simulink library "My_library"  (R2024b)
settings: Solver=VariableStepAuto  StartTime=0.0  StopTime=10.0  RelTol=1e-3
undefined symbols (not defined in the file): DiscIntNeverNeededParam, L
libraries: slpidlib x3, dspfdesign x2, eeGeneralControl x1
settings Model: Creator=sa127  LastModifiedBy=sa127

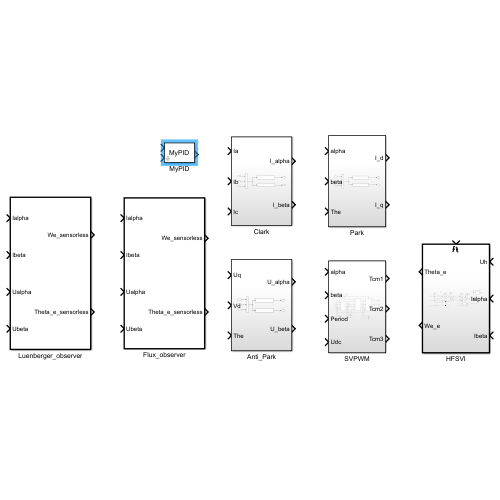
[thumbnail: Simulink's stored preview of the top-level diagram]
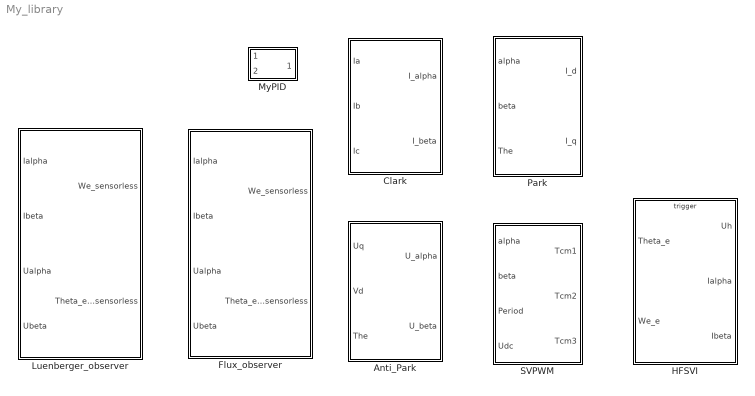
== system My_library ==
  Anti_Park : Subsystem
  Clark : Subsystem
  Flux_observer : Subsystem  TreatAsAtomicUnit=on  mask{gamma=100000, PLL_P=0, PLL_I=0, Rs=0, Ls=0, flux=0, Ts=0}
      mask prompts: gamma "磁链观测器增益"; PLL_P "锁相环Kp"; PLL_I "锁相环Ki"; Rs "电机相电阻"; Ls "电机相电感"; flux "永磁体磁链"; Ts "计算周期"
      mask DialogControl ParameterGroupVar Prompt: 参数
  HFSVI : Subsystem  TreatAsAtomicUnit=on
  Luenberger_observer : Subsystem  TreatAsAtomicUnit=on  mask{Rs=0, Ls=0, K1=0, K2=0, PLL_P=0, PLL_I=0, Ts=0}
      mask prompts: Rs "电机相电阻"; Ls "电机相电感"; K1 "增益K1"; K2 "增益K2"; PLL_P "锁相环Kp"; PLL_I "锁相环Ki"; Ts "运行周期"
      mask DialogControl ParameterGroupVar Prompt: 参数
  MyPID : Subsystem  mask{Kp=0.05, Ki=5, Kd=0, Ts=0.0001, max_Integral=500, min_Integral=-500, max_output=500, min_output=-500}
      mask prompts: max_Integral "积分上限"; min_Integral "积分下限"; max_output "输出上限"; min_output "输出下限"
      mask DialogControl DescTextVar Prompt: PID控制器
      mask DialogControl ParameterGroupVar Prompt: 参数
      mask Display: fprintf('MyPID');
  Park : Subsystem
  SVPWM : Subsystem

== system My_library/Anti_Park ==
  Uq : Inport
  Vd : Inport  Port=2
  The : Inport  Port=3
  Fcn : Fcn  Expr=cos(u(3))*u(2)-sin(u(3))*u(1)
  Fcn1 : Fcn  Expr=sin(u(3))*u(2)+cos(u(3))*u(1)
  Mux : Mux  Inputs=3
  U_alpha : Outport
  U_beta : Outport  Port=2
  wires:
  The/1 -> Mux/3
  Uq/1 -> Mux/1
  Fcn1/1 -> U_beta/1
  Vd/1 -> Mux/2
  Fcn/1 -> U_alpha/1
  Mux/1 -> Fcn/1, Fcn1/1

== system My_library/Clark ==
  Ia : Inport
  Ib : Inport  Port=2
  Ic : Inport  Port=3
  Fcn : Fcn  Expr=(u(1)-0.5*u(2)-0.5*u(3))*2/3
  Fcn1 : Fcn  Expr=(sqrt(3)/2*u(2)-sqrt(3)/2*u(3))*2/3
  Mux : Mux  Inputs=3
  I_alpha : Outport
  I_beta : Outport  Port=2
  wires:
  Ia/1 -> Mux/1
  Fcn/1 -> I_alpha/1
  Mux/1 -> Fcn/1, Fcn1/1
  Ic/1 -> Mux/3
  Fcn1/1 -> I_beta/1
  Ib/1 -> Mux/2

== system My_library/Flux_observer ==
  Ialpha : Inport
  Ibeta : Inport  Port=2
  Ualpha : Inport  Port=3
  Ubeta : Inport  Port=4
  OBSERVER : Subsystem
  PLL : Subsystem
  Scope6 : Scope  NumInputPorts=2
  We_sensorless : Outport
  Theta_e_sensorless : Outport  Port=2
  wires:
  Ibeta/1 -> OBSERVER/2(Ibeta)
  OBSERVER/1(sin) -> PLL/1(sin), Scope6/1  "sin_theta"
  OBSERVER/2(cos) -> PLL/2(cos), Scope6/2  "cos_theta"
  PLL/1(We) -> We_sensorless/1
  PLL/2(Theta_e) -> Theta_e_sensorless/1
  Ualpha/1 -> OBSERVER/3(Ualpha)
  Ubeta/1 -> OBSERVER/4(Ubeta)
  Ialpha/1 -> OBSERVER/1(Ialpha)

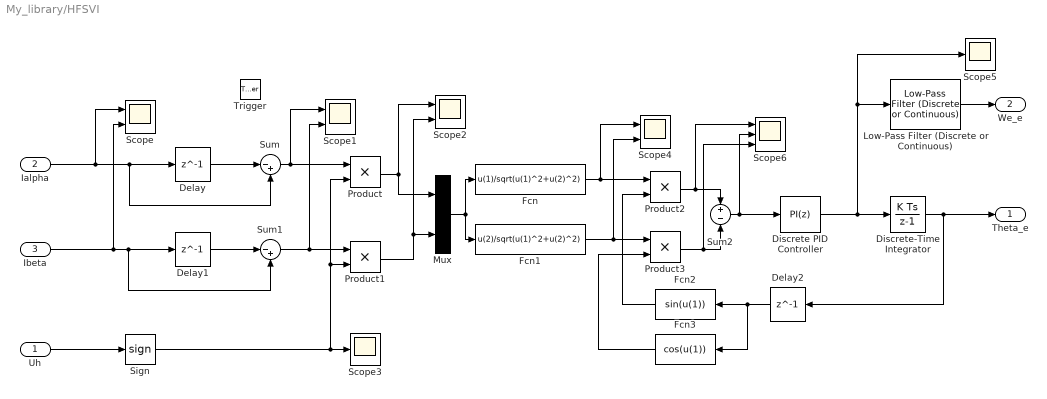
== system My_library/HFSVI ==
  Uh : Inport
  Ialpha : Inport  Port=2
  Ibeta : Inport  Port=3
  Trigger : TriggerPort  TriggerType=either  VariantControl=(inherit)
  Delay : Delay  DelayLength=1  InitialCondition=0
  Delay1 : Delay  DelayLength=1  InitialCondition=0
  Delay2 : Delay  DelayLength=1  InitialCondition=0
  Discrete PID Controller : slpidlib/PID Controller  Controller=PI  Form=Parallel  TimeDomain=Discrete-time  UseExternalTs=off  SampleTime=-1  IntegratorMethod=Forward Euler  FilterMethod=Forward Euler  ControllerParametersSource=internal  P=300  I=40000  UseKiTs=off  D=0  UseExternalDerivativeSource=off  N=100  UseFilter=on  TunerSelectOption=Transfer Function Based (PID Tuner App)  InitialConditionSource=internal  InitialConditionForIntegrator=0  InitialConditionForFilter=0  DifferentiatorICPrevScaledInput=0  ExternalReset=none  TrackingMode=off  Kt=1  LimitOutput=off  SatLimitsSource=internal  UpperSaturationLimit=inf  LowerSaturationLimit=-inf  LinearizeAsGain=off  AntiWindupMode=none  Kb=1  LimitIntegrator=off  UpperIntegratorSaturationLimit=inf  LowerIntegratorSaturationLimit=-inf  POutMin=[]  POutMax=[]  IOutMin=[]  IOutMax=[]  DOutMin=[]  DOutMax=[]  NOutMin=[]  NOutMax=[]  SumOutMin=[]  SumOutMax=[]  SaturationOutMin=[]  SaturationOutMax=[]  PParamMin=[]  PParamMax=[]  IParamMin=[]  IParamMax=[]  DParamMin=[]  DParamMax=[]  NParamMin=[]  NParamMax=[]  KbParamMin=[]  KbParamMax=[]  KtParamMin=[]  KtParamMax=[]  KbOutMin=[]  KbOutMax=[]  KtOutMin=[]  KtOutMax=[]  IntegratorOutMin=[]  IntegratorOutMax=[]  FilterOutMin=[]  FilterOutMax=[]  SumI1OutMin=[]  SumI1OutMax=[]  SumI2OutMin=[]  SumI2OutMax=[]  SumI3OutMin=[]  SumI3OutMax=[]  SumI4OutMin=[]  SumI4OutMax=[]  SumDOutMin=[]  SumDOutMax=[]  DifferentiatorOutMin=[]  DifferentiatorOutMax=[]  FilterDiffOutCoefMin=[]  FilterDiffOutCoefMax=[]  ReciprocalOutMin=[]  ReciprocalOutMax=[]  SumDenOutMin=[]  SumDenOutMax=[]  SumNumOutMin=[]  SumNumOutMax=[]  DivideOutMin=[]  DivideOutMax=[]  UdiffTsProdOutMin=[]  UdiffTsProdOutMax=[]  NTsProdOutMin=[]  NTsProdOutMax=[]  UintegralTsProdOutMin=[]  UintegralTsProdOutMax=[]  UngainTsProdOutMin=[]  UngainTsProdOutMax=[]  ClampingZeroOutDataTypeStr=Inherit: Inherit via back propagation  ClampingZeroOutMin=[]  ClampingZeroOutMax=[]  FilterDenConstantOutDataTypeStr=Inherit: Inherit via back propagation  FilterDenConstantOutMin=[]  FilterDenConstantOutMax=[]  PCopyOutDataTypeStr=Inherit: Inherit via back propagation  PCopyOutMin=[]  PCopyOutMax=[]  NCopyOutDataTypeStr=Inherit: Inherit via back propagation  NCopyOutMin=[]  NCopyOutMax=[]  IntegratorContinuousStateAttributes=''  IntegratorStateMustResolveToSignalObject=off  IntegratorRTWStateStorageClass=Auto  FilterContinuousStateAttributes=''  FilterStateMustResolveToSignalObject=off  FilterRTWStateStorageClass=Auto  ParallelPVariant=InternalParameters  IdealPVariant=Disabled  IVariant=InternalParameters  DVariant=Disabled  IntegratorVariant=Discrete  SatVariant=Disabled  AWVariant=Passthrough  PCopyVariant=Disabled  TRVariant=Disabled  FdbkBlocksVariant=Forward  IdealPFdbkVariant=Disabled  SatFdbkVariant=Disabled  DerivativeFilterVariant=Disabled  NVariant=Disabled  NCopyVariant=Disabled_SignalSpec  FilterICVariant=Disabled  IntegratorICVariant=InternalICs  ExternalResetVariant=Disabled  TRSumVariant=Passthrough  SumFdbkVariant=Disabled  SumVariant=Sum_PI  TsampFilterVariant=InternalTs  TsampNgainVariant=Passthrough  TsampIntegralVariant=Disabled_SignalSpec  ExternalSaturationOutDataTypeStr=Inherit: Same as second input  DerivativeSourceVariant=Disabled  PreIntVariant=InternalPreInt
  Discrete-Time Integrator : DiscreteIntegrator  SampleTime=-1  ICPrevOutput=DiscIntNeverNeededParam  ICPrevScaledInput=DiscIntNeverNeededParam
  Fcn : Fcn  Expr=u(1)/sqrt(u(1)^2+u(2)^2)
  Fcn1 : Fcn  Expr=u(2)/sqrt(u(1)^2+u(2)^2)
  Fcn2 : Fcn  Expr=sin(u(1))
  Fcn3 : Fcn  Expr=cos(u(1))
  Low-Pass Filter (Discrete or Continuous) : eeGeneralControl/Low-Pass Filter (Discrete or Continuous)  K=1  T=0.01  B=inf  A=-inf  init_option=Inherited from block input  x0=0  Ts=-1
  Mux : Mux  Inputs=2
  Product{,1..3} (4 alike) : Product
  Scope{,1..2,4} (4 alike) : Scope  NumInputPorts=2
  Scope3 : Scope
  Scope5 : Scope
  Scope6 : Scope  NumInputPorts=3
  Sign : Signum
  Sum : Sum  Inputs=|-+
  Sum1 : Sum  Inputs=|-+
  Sum2 : Sum  Inputs=+-
  Theta_e : Outport
  We_e : Outport  Port=2
  wires:
  Delay/1 -> Sum/1
  Delay1/1 -> Sum1/1
  Sum/1 -> Product/1, Scope1/1
  Sum1/1 -> Product1/1, Scope1/2
  Uh/1 -> Sign/1
  Sign/1 -> Scope3/1, Product1/2, Product/2
  Product/1 -> Mux/1, Scope2/1
  Product1/1 -> Mux/2, Scope2/2
  Mux/1 -> Fcn1/1, Fcn/1
  Fcn/1 -> Product2/1, Scope4/1
  Fcn1/1 -> Scope4/2, Product3/1
  Fcn2/1 -> Product2/2
  Fcn3/1 -> Product3/2
  Product2/1 -> Scope6/1, Sum2/1
  Product3/1 -> Sum2/2, Scope6/3
  Discrete PID Controller/1 -> Scope5/1, Low-Pass Filter (Discrete or Continuous)/1, Discrete-Time Integrator/1
  Delay2/1 -> Fcn3/1, Fcn2/1
  Sum2/1 -> Scope6/2, Discrete PID Controller/1
  Low-Pass Filter (Discrete or Continuous)/1 -> We_e/1
  Ialpha/1 -> Sum/2, Delay/1, Scope/1
  Ibeta/1 -> Scope/2, Sum1/2, Delay1/1
  Discrete-Time Integrator/1 -> Theta_e/1, Delay2/1

== system My_library/Luenberger_observer ==
  Ialpha : Inport
  Ibeta : Inport  Port=2
  Ualpha : Inport  Port=3
  Ubeta : Inport  Port=4
  OBSERVER : Subsystem
  PLL : Subsystem
  Scope6 : Scope  NumInputPorts=2
  We_sensorless : Outport
  Theta_e_sensorless : Outport  Port=2
  wires:
  Ibeta/1 -> OBSERVER/2(Ibeta)
  OBSERVER/1(Ealpha_hat) -> PLL/1(Ealpha_hat), Scope6/1  "sin_theta"
  OBSERVER/2(Ebeta_hat) -> PLL/2(Ebeta_hat), Scope6/2  "cos_theta"
  PLL/1(We) -> We_sensorless/1, OBSERVER/5(We)
  PLL/2(Theta_e) -> Theta_e_sensorless/1
  Ualpha/1 -> OBSERVER/3(Ualpha)
  Ubeta/1 -> OBSERVER/4(Ubeta)
  Ialpha/1 -> OBSERVER/1(Ialpha)

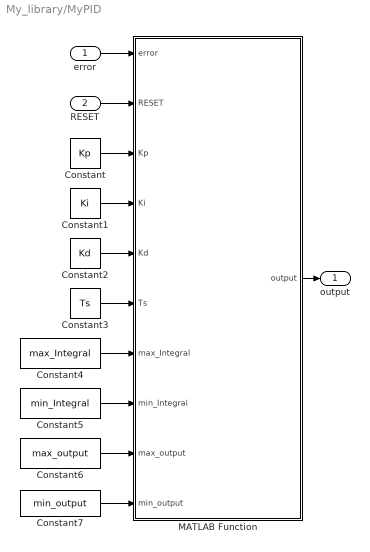
== system My_library/MyPID ==
  error : Inport
  RESET : Inport  Port=2
  Constant : Constant  Value=Kp
  Constant1 : Constant  Value=Ki
  Constant2 : Constant  Value=Kd
  Constant3 : Constant  Value=Ts
  Constant4 : Constant  Value=max_Integral
  Constant5 : Constant  Value=min_Integral
  Constant6 : Constant  Value=max_output
  Constant7 : Constant  Value=min_output
  MATLAB Function : MATLAB Function  TreatAsAtomicUnit=on
  output : Outport
  wires:
  MATLAB Function/1(output) -> output/1
  Constant2/1 -> MATLAB Function/5(Kd)
  Constant6/1 -> MATLAB Function/9(max_output)
  Constant1/1 -> MATLAB Function/4(Ki)
  error/1 -> MATLAB Function/1(error)
  Constant5/1 -> MATLAB Function/8(min_Integral)
  Constant4/1 -> MATLAB Function/7(max_Integral)
  Constant/1 -> MATLAB Function/3(Kp)
  Constant7/1 -> MATLAB Function/10(min_output)
  Constant3/1 -> MATLAB Function/6(Ts)
  RESET/1 -> MATLAB Function/2(RESET)

== system My_library/Park ==
  alpha : Inport
  beta : Inport  Port=2
  The : Inport  Port=3
  Fcn : Fcn  Expr=cos(u(3))*u(1)+sin(u(3))*u(2)
  Fcn1 : Fcn  Expr=-sin(u(3))*u(1)+cos(u(3))*u(2)
  Mux : Mux  Inputs=3
  I_d : Outport
  I_q : Outport  Port=2
  wires:
  beta/1 -> Mux/2
  Mux/1 -> Fcn/1, Fcn1/1
  alpha/1 -> Mux/1
  The/1 -> Mux/3
  Fcn1/1 -> I_q/1
  Fcn/1 -> I_d/1

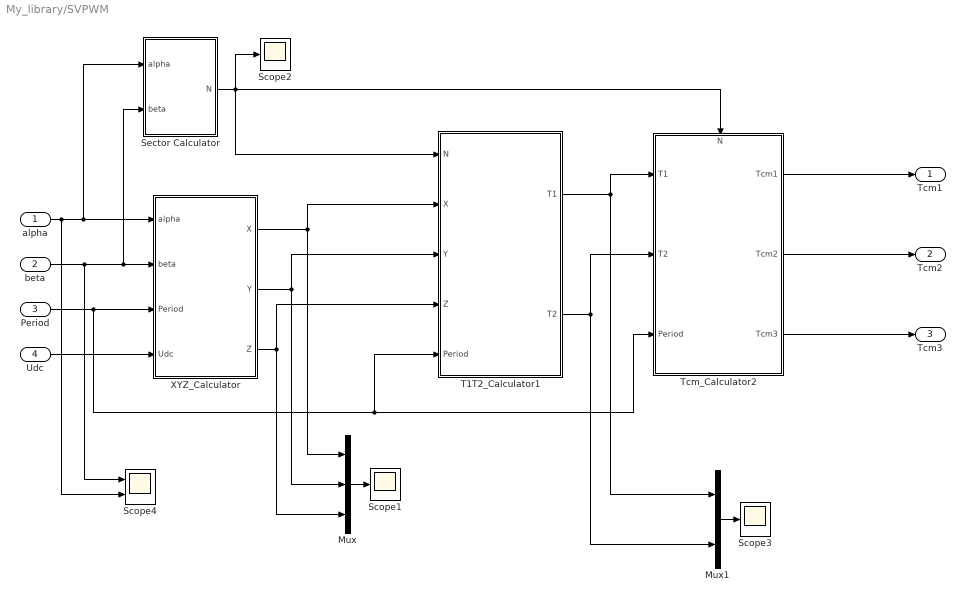
== system My_library/SVPWM ==
  alpha : Inport
  beta : Inport  Port=2
  Period : Inport  Port=3
  Udc : Inport  Port=4
  Mux : Mux  Inputs=3
  Mux1 : Mux  Inputs=2
  Scope1 : Scope
  Scope2 : Scope
  Scope3 : Scope
  Scope4 : Scope  NumInputPorts=2
  Sector Calculator : Subsystem
  T1T2_Calculator1 : Subsystem
  Tcm_Calculator2 : Subsystem
      settings: PortSchema="{\"entries\":[{\"content\":{\"sides\":[{\"content\":{\"connectorIds\":[\"In1\",\"In2\",\"In3\"]},\"type\":\"ConnectorPlacement.EquallySpacedRectSide\",\"uuid\":\"6148b169-7250-44a2-b567-24c78ff320ed\"},{\"content\":{\"connectorIds\":[\"Out1\",\"Out2\",\"Out3\"],\"side\":\"RIGHT\"},\"type\":\"ConnectorPlacement.EquallySpacedRectSide\",\"uuid\":\"6efb5841-0c91-46f1-a519-7a6c3f211abe\"},{\"content\":{\"connectorIds\":[\"In4\"],\"side\":\"TOP\"},\"type\":\"ConnectorPlacement.EquallySpacedRectSide\",\"uuid\":\"038beb55-4291-4f93-808f-b37c10172b21\"}]},\"type\":\"ConnectorPlacement.EquallySpacedConnector\",\"uuid\":\"c2a58b65-6aee-438a-88be-c8e96908c0e6\"}],\"packageUris\":[\"http://schema.mathworks.com/mf0/Connector/R2020b\"],\"version\":\"1.0\"}"
  XYZ_Calculator : Subsystem
  Tcm1 : Outport
  Tcm2 : Outport  Port=2
  Tcm3 : Outport  Port=3
  wires:
  XYZ_Calculator/1(X) -> T1T2_Calculator1/2(X), Mux/1
  Period/1 -> Tcm_Calculator2/3(Period), T1T2_Calculator1/5(Period), XYZ_Calculator/3(Period)
  Tcm_Calculator2/1(Tcm1) -> Tcm1/1
  XYZ_Calculator/3(Z) -> T1T2_Calculator1/4(Z), Mux/3
  Mux1/1 -> Scope3/1
  Udc/1 -> XYZ_Calculator/4(Udc)
  Sector Calculator/1(N) -> T1T2_Calculator1/1(N), Tcm_Calculator2/4(N), Scope2/1
  XYZ_Calculator/2(Y) -> T1T2_Calculator1/3(Y), Mux/2
  alpha/1 -> Scope4/2, XYZ_Calculator/1(alpha), Sector Calculator/1(alpha)
  beta/1 -> Scope4/1, XYZ_Calculator/2(beta), Sector Calculator/2(beta)
  T1T2_Calculator1/2(T2) -> Tcm_Calculator2/2(T2), Mux1/2
  T1T2_Calculator1/1(T1) -> Tcm_Calculator2/1(T1), Mux1/1
  Mux/1 -> Scope1/1
  Tcm_Calculator2/3(Tcm3) -> Tcm3/1
  Tcm_Calculator2/2(Tcm2) -> Tcm2/1

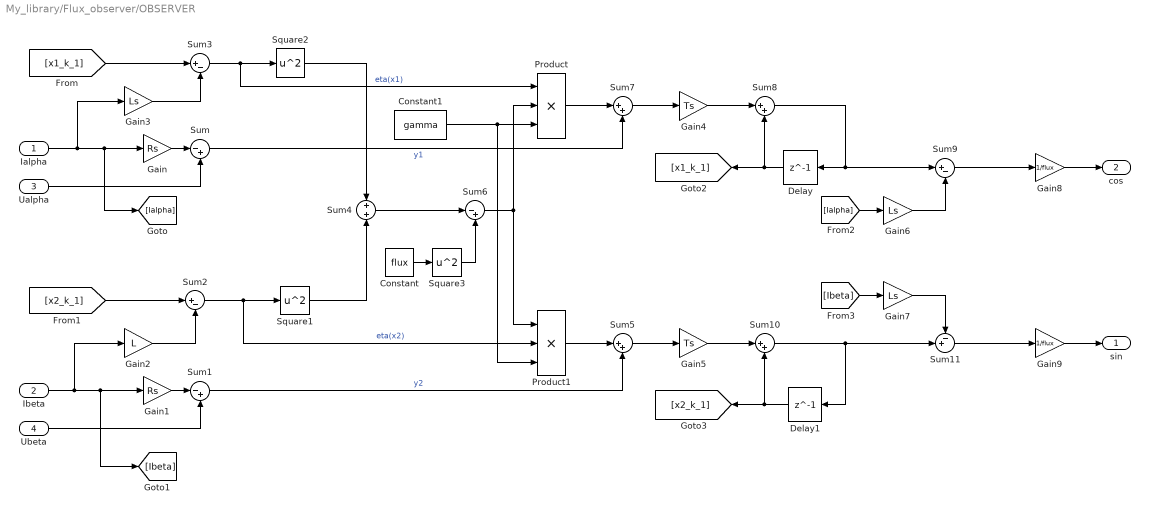
== system My_library/Flux_observer/OBSERVER ==
  Ialpha : Inport
  Ibeta : Inport  Port=2
  Ualpha : Inport  Port=3
  Ubeta : Inport  Port=4
  Constant : Constant  Value=flux
  Constant1 : Constant  Value=gamma
  Delay : Delay  DelayLength=1  InputProcessing=Columns as channels (frame based)
  Delay1 : Delay  DelayLength=1  InputProcessing=Columns as channels (frame based)
  Gain : Gain  Gain=Rs
  Gain1 : Gain  Gain=Rs
  Gain2 : Gain  Gain=L
  Gain3 : Gain  Gain=Ls
  Gain4 : Gain  Gain=Ts
  Gain5 : Gain  Gain=Ts
  Gain6 : Gain  Gain=Ls
  Gain7 : Gain  Gain=Ls
  Gain8 : Gain  Gain=1/flux
  Gain9 : Gain  Gain=1/flux
  Product : Product  Inputs=3
  Product1 : Product  Inputs=3
  Square1 : Math  Operator=square
  Square2 : Math  Operator=square
  Square3 : Math  Operator=square
  Sum : Sum  Inputs=|-+
  Sum1 : Sum  Inputs=|-+
  Sum{5,7..8,10} (4 alike) : Sum  Inputs=|++
  Sum11 : Sum  Inputs=-+|
  Sum2 : Sum  Inputs=|+-
  Sum3 : Sum  Inputs=|+-
  Sum4 : Sum
  Sum6 : Sum  Inputs=|-+
  Sum9 : Sum  Inputs=|+-
  sin : Outport
  cos : Outport  Port=2
  wires:
  Ialpha/1 -> Gain3/1, [Ialpha], Gain/1
  Gain/1 -> Sum/1
  Ualpha/1 -> Sum/2
  Ubeta/1 -> Sum1/2
  Gain1/1 -> Sum1/1
  Ibeta/1 -> Gain2/1, [Ibeta], Gain1/1
  Sum1/1 -> Sum5/2  "y2"
  Sum/1 -> Sum7/2  "y1"
  [x2_k_1] -> Sum2/1
  [x1_k_1] -> Sum3/1
  Gain2/1 -> Sum2/2
  Gain3/1 -> Sum3/2
  Sum3/1 -> Product/1, Square2/1  "eta(x1)"
  Sum2/1 -> Product1/2, Square1/1  "eta(x2)"
  Square2/1 -> Sum4/1
  Square1/1 -> Sum4/2
  Sum4/1 -> Sum6/1
  Square3/1 -> Sum6/2
  Constant/1 -> Square3/1
  Sum6/1 -> Product1/1, Product/2
  Constant1/1 -> Product1/3, Product/3
  Product1/1 -> Sum5/1
  Product/1 -> Sum7/1
  Sum5/1 -> Gain5/1
  Sum7/1 -> Gain4/1
  Sum8/1 -> Sum9/1, Delay/1
  Delay/1 -> [x1_k_1], Sum8/2
  Gain4/1 -> Sum8/1
  Sum10/1 -> Sum11/2, Delay1/1
  Delay1/1 -> [x2_k_1], Sum10/2
  Gain5/1 -> Sum10/1
  [Ialpha] -> Gain6/1
  [Ibeta] -> Gain7/1
  Gain6/1 -> Sum9/2
  Gain7/1 -> Sum11/1
  Sum9/1 -> Gain8/1
  Gain8/1 -> cos/1
  Gain9/1 -> sin/1
  Sum11/1 -> Gain9/1

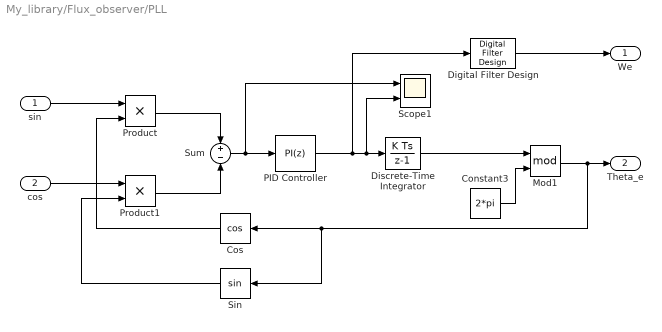
== system My_library/Flux_observer/PLL ==
  sin : Inport
  cos : Inport  Port=2
  Constant3 : Constant  Value=2*pi
  Cos : Trigonometry  Operator=cos  ApproximationMethod=Lookup
  Digital Filter Design : dspfdesign/Digital Filter Design  mwdsp_browser_bugfix_var=off
  Discrete-Time Integrator : DiscreteIntegrator  SampleTime=-1  ICPrevOutput=DiscIntNeverNeededParam  ICPrevScaledInput=DiscIntNeverNeededParam
  Mod1 : Math  Operator=mod
  PID Controller : slpidlib/PID Controller  Controller=PI  Form=Parallel  TimeDomain=Discrete-time  UseExternalTs=off  SampleTime=-1  IntegratorMethod=Forward Euler  FilterMethod=Forward Euler  ControllerParametersSource=internal  P=PLL_P  I=PLL_I  UseKiTs=off  D=0  UseExternalDerivativeSource=off  N=100  UseFilter=on  TunerSelectOption=Transfer Function Based (PID Tuner App)  InitialConditionSource=internal  InitialConditionForIntegrator=0  InitialConditionForFilter=0  DifferentiatorICPrevScaledInput=0  ExternalReset=none  TrackingMode=off  Kt=1  LimitOutput=off  SatLimitsSource=internal  UpperSaturationLimit=inf  LowerSaturationLimit=-inf  LinearizeAsGain=on  AntiWindupMode=none  Kb=1  LimitIntegrator=off  UpperIntegratorSaturationLimit=100000  LowerIntegratorSaturationLimit=-100000  POutMin=[]  POutMax=[]  IOutMin=[]  IOutMax=[]  DOutMin=[]  DOutMax=[]  NOutMin=[]  NOutMax=[]  SumOutMin=[]  SumOutMax=[]  SaturationOutMin=[]  SaturationOutMax=[]  PParamMin=[]  PParamMax=[]  IParamMin=[]  IParamMax=[]  DParamMin=[]  DParamMax=[]  NParamMin=[]  NParamMax=[]  KbParamMin=[]  KbParamMax=[]  KtParamMin=[]  KtParamMax=[]  KbOutMin=[]  KbOutMax=[]  KtOutMin=[]  KtOutMax=[]  IntegratorOutMin=[]  IntegratorOutMax=[]  FilterOutMin=[]  FilterOutMax=[]  SumI1OutMin=[]  SumI1OutMax=[]  SumI2OutMin=[]  SumI2OutMax=[]  SumI3OutMin=[]  SumI3OutMax=[]  SumI4OutMin=[]  SumI4OutMax=[]  SumDOutMin=[]  SumDOutMax=[]  DifferentiatorOutMin=[]  DifferentiatorOutMax=[]  FilterDiffOutCoefMin=[]  FilterDiffOutCoefMax=[]  ReciprocalOutMin=[]  ReciprocalOutMax=[]  SumDenOutMin=[]  SumDenOutMax=[]  SumNumOutMin=[]  SumNumOutMax=[]  DivideOutMin=[]  DivideOutMax=[]  UdiffTsProdOutMin=[]  UdiffTsProdOutMax=[]  NTsProdOutMin=[]  NTsProdOutMax=[]  UintegralTsProdOutMin=[]  UintegralTsProdOutMax=[]  UngainTsProdOutMin=[]  UngainTsProdOutMax=[]  ClampingZeroOutDataTypeStr=Inherit: Inherit via back propagation  ClampingZeroOutMin=[]  ClampingZeroOutMax=[]  FilterDenConstantOutDataTypeStr=Inherit: Inherit via back propagation  FilterDenConstantOutMin=[]  FilterDenConstantOutMax=[]  PCopyOutDataTypeStr=Inherit: Inherit via back propagation  PCopyOutMin=[]  PCopyOutMax=[]  NCopyOutDataTypeStr=Inherit: Inherit via back propagation  NCopyOutMin=[]  NCopyOutMax=[]  IntegratorContinuousStateAttributes=''  IntegratorStateMustResolveToSignalObject=off  IntegratorRTWStateStorageClass=Auto  FilterContinuousStateAttributes=''  FilterStateMustResolveToSignalObject=off  FilterRTWStateStorageClass=Auto  ParallelPVariant=InternalParameters  IdealPVariant=Disabled  IVariant=InternalParameters  DVariant=Disabled  IntegratorVariant=Discrete  SatVariant=Disabled  AWVariant=Passthrough  PCopyVariant=Disabled  TRVariant=Disabled  FdbkBlocksVariant=Forward  IdealPFdbkVariant=Disabled  SatFdbkVariant=Disabled  DerivativeFilterVariant=Disabled  NVariant=Disabled  NCopyVariant=Disabled_SignalSpec  FilterICVariant=Disabled  IntegratorICVariant=InternalICs  ExternalResetVariant=Disabled  TRSumVariant=Passthrough  SumFdbkVariant=Disabled  SumVariant=Sum_PI  TsampFilterVariant=InternalTs  TsampNgainVariant=Passthrough  TsampIntegralVariant=Disabled_SignalSpec  ExternalSaturationOutDataTypeStr=Inherit: Same as second input  DerivativeSourceVariant=Disabled  PreIntVariant=InternalPreInt
  Product : Product
  Product1 : Product
  Scope1 : Scope  NumInputPorts=2
  Sin : Trigonometry  ApproximationMethod=Lookup
  Sum : Sum  Inputs=+-
  We : Outport
  Theta_e : Outport  Port=2
  wires:
  Mod1/1 -> Sin/1, Cos/1, Theta_e/1
  Constant3/1 -> Mod1/2
  PID Controller/1 -> Digital Filter Design/1, Scope1/2, Discrete-Time Integrator/1
  Sin/1 -> Product1/2
  Cos/1 -> Product/2
  Product/1 -> Sum/1
  Product1/1 -> Sum/2
  Discrete-Time Integrator/1 -> Mod1/1
  Sum/1 -> Scope1/1, PID Controller/1
  sin/1 -> Product/1
  cos/1 -> Product1/1
  Digital Filter Design/1 -> We/1

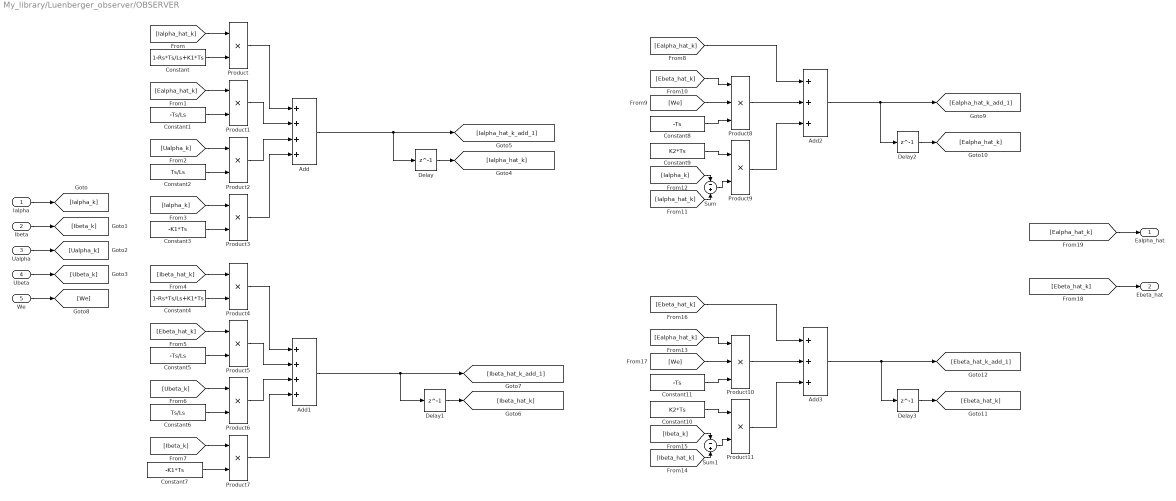
== system My_library/Luenberger_observer/OBSERVER ==
  Ialpha : Inport
  Ibeta : Inport  Port=2
  Ualpha : Inport  Port=3
  Ubeta : Inport  Port=4
  We : Inport  Port=5
  Add : Sum  Inputs=++++
  Add1 : Sum  Inputs=++++
  Add2 : Sum  Inputs=+++
  Add3 : Sum  Inputs=+++
  Constant : Constant  Value=1-Rs*Ts/Ls+K1*Ts
  Constant1 : Constant  Value=-Ts/Ls
  Constant10 : Constant  Value=K2*Ts
  Constant11 : Constant  Value=-Ts
  Constant2 : Constant  Value=Ts/Ls
  Constant3 : Constant  Value=-K1*Ts
  Constant4 : Constant  Value=1-Rs*Ts/Ls+K1*Ts
  Constant5 : Constant  Value=-Ts/Ls
  Constant6 : Constant  Value=Ts/Ls
  Constant7 : Constant  Value=-K1*Ts
  Constant8 : Constant  Value=-Ts
  Constant9 : Constant  Value=K2*Ts
  Delay{,1..3} (4 alike) : Delay  DelayLength=1  InputProcessing=Columns as channels (frame based)
  Product{,1..7,9,11} (10 alike) : Product
  Product10 : Product  Inputs=3
  Product8 : Product  Inputs=3
  Sum : Sum  Inputs=-+
  Sum1 : Sum  Inputs=-+
  Ealpha_hat : Outport
  Ebeta_hat : Outport  Port=2
  wires:
  [Ialpha_hat_k] -> Product/1
  Constant/1 -> Product/2
  Product/1 -> Add/1
  [Ealpha_hat_k] -> Product1/1
  Constant1/1 -> Product1/2
  Constant2/1 -> Product2/2
  [Ualpha_k] -> Product2/1
  [Ialpha_k] -> Product3/1
  Constant3/1 -> Product3/2
  Product1/1 -> Add/2
  Product2/1 -> Add/3
  Product3/1 -> Add/4
  Ialpha/1 -> [Ialpha_k]
  Ubeta/1 -> [Ubeta_k]
  Ualpha/1 -> [Ualpha_k]
  Ibeta/1 -> [Ibeta_k]
  Delay/1 -> [Ialpha_hat_k]
  Delay1/1 -> [Ibeta_hat_k]
  [Ibeta_hat_k] -> Product4/1
  [Ibeta_k] -> Product7/1
  Constant7/1 -> Product7/2
  Constant5/1 -> Product5/2
  [Ebeta_hat_k] -> Product5/1
  Product6/1 -> Add1/3
  Product5/1 -> Add1/2
  [Ubeta_k] -> Product6/1
  Constant6/1 -> Product6/2
  Product7/1 -> Add1/4
  Constant4/1 -> Product4/2
  Product4/1 -> Add1/1
  We/1 -> [We]
  [We] -> Product8/2
  Constant8/1 -> Product8/3
  [Ebeta_hat_k] -> Product8/1
  [Ialpha_k] -> Sum/1
  [Ialpha_hat_k] -> Sum/2
  Constant9/1 -> Product9/1
  Sum/1 -> Product9/2
  Product9/1 -> Add2/3
  Delay2/1 -> [Ealpha_hat_k]
  [Ealpha_hat_k] -> Product10/1
  Constant11/1 -> Product10/3
  [Ebeta_hat_k] -> Add3/1
  [Ibeta_k] -> Sum1/1
  [We] -> Product10/2
  [Ibeta_hat_k] -> Sum1/2
  Delay3/1 -> [Ebeta_hat_k]
  Sum1/1 -> Product11/2
  Constant10/1 -> Product11/1
  Product11/1 -> Add3/3
  [Ealpha_hat_k] -> Ealpha_hat/1
  [Ebeta_hat_k] -> Ebeta_hat/1
  Product10/1 -> Add3/2
  Add/1 -> Delay/1, [Ialpha_hat_k_add_1]
  Add1/1 -> Delay1/1, [Ibeta_hat_k_add_1]
  Product8/1 -> Add2/2
  [Ealpha_hat_k] -> Add2/1
  Add3/1 -> Delay3/1, [Ebeta_hat_k_add_1]
  Add2/1 -> Delay2/1, [Ealpha_hat_k_add_1]

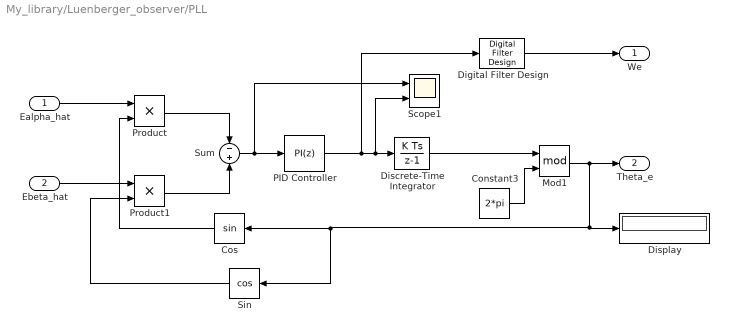
== system My_library/Luenberger_observer/PLL ==
  Ealpha_hat : Inport
  Ebeta_hat : Inport  Port=2
  Constant3 : Constant  Value=2*pi
  Cos : Trigonometry  NumberOfIterations=20
  Digital Filter Design : dspfdesign/Digital Filter Design  mwdsp_browser_bugfix_var=off
  Discrete-Time Integrator : DiscreteIntegrator  SampleTime=-1  ICPrevOutput=DiscIntNeverNeededParam  ICPrevScaledInput=DiscIntNeverNeededParam
  Display : Display
  Mod1 : Math  Operator=mod
  PID Controller : slpidlib/PID Controller  Controller=PI  Form=Parallel  TimeDomain=Discrete-time  UseExternalTs=off  SampleTime=-1  IntegratorMethod=Forward Euler  FilterMethod=Forward Euler  ControllerParametersSource=internal  P=PLL_P  I=PLL_I  UseKiTs=off  D=0  UseExternalDerivativeSource=off  N=100  UseFilter=on  TunerSelectOption=Transfer Function Based (PID Tuner App)  InitialConditionSource=internal  InitialConditionForIntegrator=0  InitialConditionForFilter=0  DifferentiatorICPrevScaledInput=0  ExternalReset=none  TrackingMode=off  Kt=1  LimitOutput=off  SatLimitsSource=internal  UpperSaturationLimit=inf  LowerSaturationLimit=-inf  LinearizeAsGain=on  AntiWindupMode=none  Kb=1  LimitIntegrator=off  UpperIntegratorSaturationLimit=100000  LowerIntegratorSaturationLimit=-100000  POutMin=[]  POutMax=[]  IOutMin=[]  IOutMax=[]  DOutMin=[]  DOutMax=[]  NOutMin=[]  NOutMax=[]  SumOutMin=[]  SumOutMax=[]  SaturationOutMin=[]  SaturationOutMax=[]  PParamMin=[]  PParamMax=[]  IParamMin=[]  IParamMax=[]  DParamMin=[]  DParamMax=[]  NParamMin=[]  NParamMax=[]  KbParamMin=[]  KbParamMax=[]  KtParamMin=[]  KtParamMax=[]  KbOutMin=[]  KbOutMax=[]  KtOutMin=[]  KtOutMax=[]  IntegratorOutMin=[]  IntegratorOutMax=[]  FilterOutMin=[]  FilterOutMax=[]  SumI1OutMin=[]  SumI1OutMax=[]  SumI2OutMin=[]  SumI2OutMax=[]  SumI3OutMin=[]  SumI3OutMax=[]  SumI4OutMin=[]  SumI4OutMax=[]  SumDOutMin=[]  SumDOutMax=[]  DifferentiatorOutMin=[]  DifferentiatorOutMax=[]  FilterDiffOutCoefMin=[]  FilterDiffOutCoefMax=[]  ReciprocalOutMin=[]  ReciprocalOutMax=[]  SumDenOutMin=[]  SumDenOutMax=[]  SumNumOutMin=[]  SumNumOutMax=[]  DivideOutMin=[]  DivideOutMax=[]  UdiffTsProdOutMin=[]  UdiffTsProdOutMax=[]  NTsProdOutMin=[]  NTsProdOutMax=[]  UintegralTsProdOutMin=[]  UintegralTsProdOutMax=[]  UngainTsProdOutMin=[]  UngainTsProdOutMax=[]  ClampingZeroOutDataTypeStr=Inherit: Inherit via back propagation  ClampingZeroOutMin=[]  ClampingZeroOutMax=[]  FilterDenConstantOutDataTypeStr=Inherit: Inherit via back propagation  FilterDenConstantOutMin=[]  FilterDenConstantOutMax=[]  PCopyOutDataTypeStr=Inherit: Inherit via back propagation  PCopyOutMin=[]  PCopyOutMax=[]  NCopyOutDataTypeStr=Inherit: Inherit via back propagation  NCopyOutMin=[]  NCopyOutMax=[]  IntegratorContinuousStateAttributes=''  IntegratorStateMustResolveToSignalObject=off  IntegratorRTWStateStorageClass=Auto  FilterContinuousStateAttributes=''  FilterStateMustResolveToSignalObject=off  FilterRTWStateStorageClass=Auto  ParallelPVariant=InternalParameters  IdealPVariant=Disabled  IVariant=InternalParameters  DVariant=Disabled  IntegratorVariant=Discrete  SatVariant=Disabled  AWVariant=Passthrough  PCopyVariant=Disabled  TRVariant=Disabled  FdbkBlocksVariant=Forward  IdealPFdbkVariant=Disabled  SatFdbkVariant=Disabled  DerivativeFilterVariant=Disabled  NVariant=Disabled  NCopyVariant=Disabled_SignalSpec  FilterICVariant=Disabled  IntegratorICVariant=InternalICs  ExternalResetVariant=Disabled  TRSumVariant=Passthrough  SumFdbkVariant=Disabled  SumVariant=Sum_PI  TsampFilterVariant=InternalTs  TsampNgainVariant=Passthrough  TsampIntegralVariant=Disabled_SignalSpec  ExternalSaturationOutDataTypeStr=Inherit: Same as second input  DerivativeSourceVariant=Disabled  PreIntVariant=InternalPreInt
  Product : Product
  Product1 : Product
  Scope1 : Scope  NumInputPorts=2
  Sin : Trigonometry  Operator=cos  NumberOfIterations=20
  Sum : Sum  Inputs=-+
  We : Outport
  Theta_e : Outport  Port=2
  wires:
  Mod1/1 -> Theta_e/1, Display/1, Sin/1, Cos/1
  Constant3/1 -> Mod1/2
  PID Controller/1 -> Digital Filter Design/1, Scope1/2, Discrete-Time Integrator/1
  Sin/1 -> Product1/2
  Cos/1 -> Product/2
  Product/1 -> Sum/1
  Product1/1 -> Sum/2
  Discrete-Time Integrator/1 -> Mod1/1
  Sum/1 -> Scope1/1, PID Controller/1
  Ebeta_hat/1 -> Product1/1
  Digital Filter Design/1 -> We/1
  Ealpha_hat/1 -> Product/1

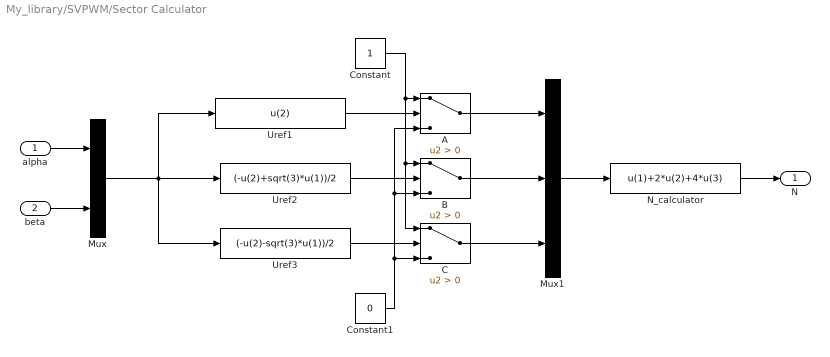
== system My_library/SVPWM/Sector Calculator ==
  alpha : Inport
  beta : Inport  Port=2
  A : Switch  Criteria=u2 > Threshold  SaturateOnIntegerOverflow=off  InputSameDT=off
  B : Switch  Criteria=u2 > Threshold  SaturateOnIntegerOverflow=off  InputSameDT=off
  C : Switch  Criteria=u2 > Threshold  SaturateOnIntegerOverflow=off  InputSameDT=off
  Constant : Constant
  Constant1 : Constant  Value=0
  Mux : Mux  Inputs=2
  Mux1 : Mux  Inputs=3
  N_calculator : Fcn  Expr=u(1)+2*u(2)+4*u(3)
  Uref1 : Fcn  Expr=u(2)
  Uref2 : Fcn  Expr=(-u(2)+sqrt(3)*u(1))/2
  Uref3 : Fcn  Expr=(-u(2)-sqrt(3)*u(1))/2
  N : Outport
  wires:
  N_calculator/1 -> N/1
  Mux1/1 -> N_calculator/1
  C/1 -> Mux1/3
  A/1 -> Mux1/1
  B/1 -> Mux1/2
  Constant1/1 -> C/3, B/3, A/3
  Constant/1 -> A/1, B/1, C/1
  Uref2/1 -> B/2
  Uref3/1 -> C/2
  alpha/1 -> Mux/1
  Uref1/1 -> A/2
  Mux/1 -> Uref1/1, Uref2/1, Uref3/1
  beta/1 -> Mux/2

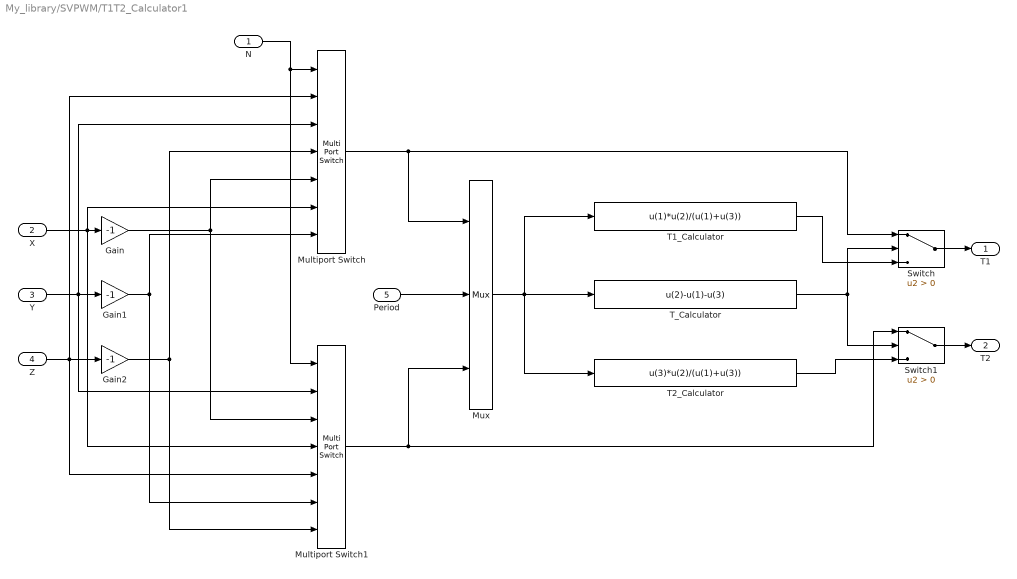
== system My_library/SVPWM/T1T2_Calculator1 ==
  N : Inport
  X : Inport  Port=2
  Y : Inport  Port=3
  Z : Inport  Port=4
  Period : Inport  Port=5
  Gain : Gain  Gain=-1
  Gain1 : Gain  Gain=-1
  Gain2 : Gain  Gain=-1
  Multiport Switch : MultiPortSwitch  Inputs=6  SaturateOnIntegerOverflow=off  InputSameDT=off
  Multiport Switch1 : MultiPortSwitch  Inputs=6  SaturateOnIntegerOverflow=off  InputSameDT=off
  Mux : Mux  Inputs=3
  Switch : Switch  Criteria=u2 > Threshold  SaturateOnIntegerOverflow=off  InputSameDT=off
  Switch1 : Switch  Criteria=u2 > Threshold  SaturateOnIntegerOverflow=off  InputSameDT=off
  T1_Calculator : Fcn  Expr=u(1)*u(2)/(u(1)+u(3))
  T2_Calculator : Fcn  Expr=u(3)*u(2)/(u(1)+u(3))
  T_Calculator : Fcn  Expr=u(2)-u(1)-u(3)
  T1 : Outport
  T2 : Outport  Port=2
  wires:
  Switch/1 -> T1/1
  Switch1/1 -> T2/1
  T2_Calculator/1 -> Switch1/3
  T1_Calculator/1 -> Switch/3
  T_Calculator/1 -> Switch/2, Switch1/2
  Mux/1 -> T_Calculator/1, T1_Calculator/1, T2_Calculator/1
  Multiport Switch1/1 -> Mux/3, Switch1/1
  Multiport Switch/1 -> Mux/1, Switch/1
  Period/1 -> Mux/2
  Gain1/1 -> Multiport Switch1/6, Multiport Switch/7
  Gain2/1 -> Multiport Switch/4, Multiport Switch1/7
  Gain/1 -> Multiport Switch/5, Multiport Switch1/3
  Z/1 -> Gain2/1, Multiport Switch/2, Multiport Switch1/5
  Y/1 -> Gain1/1, Multiport Switch/3, Multiport Switch1/2
  N/1 -> Multiport Switch1/1, Multiport Switch/1
  X/1 -> Gain/1, Multiport Switch/6, Multiport Switch1/4

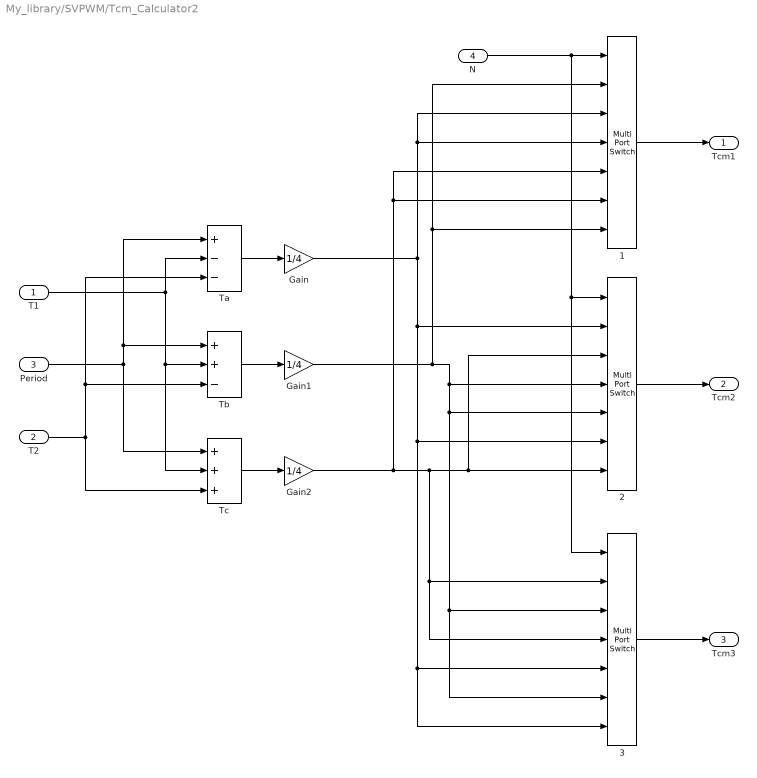
== system My_library/SVPWM/Tcm_Calculator2 ==
  T1 : Inport
  T2 : Inport  Port=2
  Period : Inport  Port=3
  N : Inport  Port=4
  1 : MultiPortSwitch  Inputs=6  SaturateOnIntegerOverflow=off  InputSameDT=off
  2 : MultiPortSwitch  Inputs=6  SaturateOnIntegerOverflow=off  InputSameDT=off
  3 : MultiPortSwitch  Inputs=6  SaturateOnIntegerOverflow=off  InputSameDT=off
  Gain : Gain  Gain=1/4
  Gain1 : Gain  Gain=1/4
  Gain2 : Gain  Gain=1/4
  Ta : Sum  Inputs=+--
  Tb : Sum  Inputs=++-
  Tc : Sum  Inputs=+++
  Tcm1 : Outport
  Tcm2 : Outport  Port=2
  Tcm3 : Outport  Port=3
  wires:
  3/1 -> Tcm3/1
  2/1 -> Tcm2/1
  1/1 -> Tcm1/1
  Gain2/1 -> 1/5, 1/6, 3/2, 3/4, 2/3, 2/7
  Gain1/1 -> 3/3, 3/6, 2/5, 2/4, 1/7, 1/2
  Gain/1 -> 1/3, 1/4, 2/2, 2/6, 3/5, 3/7
  Tc/1 -> Gain2/1
  Ta/1 -> Gain/1
  Tb/1 -> Gain1/1
  N/1 -> 1/1, 3/1, 2/1
  T2/1 -> Tc/3, Ta/3, Tb/3
  T1/1 -> Tb/2, Tc/2, Ta/2
  Period/1 -> Tc/1, Ta/1, Tb/1

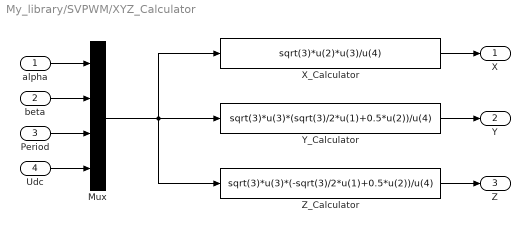
== system My_library/SVPWM/XYZ_Calculator ==
  alpha : Inport
  beta : Inport  Port=2
  Period : Inport  Port=3
  Udc : Inport  Port=4
  Mux : Mux
  X_Calculator : Fcn  Expr=sqrt(3)*u(2)*u(3)/u(4)
  Y_Calculator : Fcn  Expr=sqrt(3)*u(3)*(sqrt(3)/2*u(1)+0.5*u(2))/u(4)
  Z_Calculator : Fcn  Expr=sqrt(3)*u(3)*(-sqrt(3)/2*u(1)+0.5*u(2))/u(4)
  X : Outport
  Y : Outport  Port=2
  Z : Outport  Port=3
  wires:
  Z_Calculator/1 -> Z/1
  Y_Calculator/1 -> Y/1
  X_Calculator/1 -> X/1
  alpha/1 -> Mux/1
  Mux/1 -> X_Calculator/1, Y_Calculator/1, Z_Calculator/1
  beta/1 -> Mux/2
  Udc/1 -> Mux/4
  Period/1 -> Mux/3

== matlab function My_library/MyPID/MATLAB Function ==
  data: error input; RESET input; output output; Kp input; Ki input; Kd input; Ts input; max_Integral input; min_Integral input; max_output input; min_output input
function output = fcn(error,RESET, Kp, Ki, Kd, Ts, max_Integral, min_Integral, max_output, min_output)
%定义参数
persistent last_error;
persistent I;
persistent LAST_RESET;
% 初始化静态变量（仅在第一次调用时执行）
if isempty(last_error)
last_error = 0;  % 假设初始误差为0
end
if isempty(I)
I = 0;           % 假设初始积分项为0
end
if isempty(LAST_RESET)
LAST_RESET = 0;  % 假设初始状态为0
end

%比例项
P = Kp*error;

%积分项
I = I + Ki*error*Ts;
%积分限幅
if(I>=max_Integral)
    I = max_Integral;
elseif(I<=min_Integral)
    I = min_Integral;
end

%微分项
D = Kd*(error - last_error)/Ts;

%保留此次错误值
last_error = error;

%输出限幅
output = P+I+D;
if(output>=max_output)
    output = max_output;
elseif(output<=min_output)
    output = min_output;
end

if RESET ~= LAST_RESET
    I = 0;
    output = 0; 
end

LAST_RESET = RESET;
